simulink model "B4_quadcopter_model_discrete"  (R2021b)
settings: Solver=VariableStepAuto  StartTime=0.0  StopTime=10  FixedStep=0.002  RelTol=1e-3
values from neighbouring files (symbols this model uses):
  coef_sim_1 = tf_des_d.Denominator{1}(2)    [A11_setup_script_pprz.m]    (also in A1_setup_script.m; A6_slow_actuator.m)
  coef_sim_2 = tf_des_d.Numerator{1}(2)    [A11_setup_script_pprz.m]    (also in A1_setup_script.m; A6_slow_actuator.m)
  doublet_mag = - 0.15    (= -0.15)    [A11_setup_script_pprz.m]    (also in A1_setup_script.m)
  doublet_time = 6    [A11_setup_script_pprz.m]    (also in A1_setup_script.m)
  f_8 = 1    [A11_setup_script_pprz.m]    (also in A1_setup_script.m)
  FILT_CUTOFF = 2*pi*5    (= 31.4159265359)    [A11_setup_script_pprz.m]    (also in A1_setup_script.m)
  FILTER = 1    [A11_setup_script_pprz.m]    (also in A1_setup_script.m)
  G1 = inv(I)*G1_r    [A10_simple_plant.m]    (also in A11_setup_script_pprz.m = G1/scale; A1_setup_script.m = [G1;G1_T])
  G1_simple = inv(I)*G1_r_simple    [A1_setup_script.m]
  G2 = G2/scale    [A11_setup_script_pprz.m]    (also in A1_setup_script.m = (1/sampling_time)*inv(I)*(G2_r))
  h_plate = 0.3    [A11_setup_script_pprz.m]    (also in A1_setup_script.m = 0.16)
  I = eye(3,3)    [A10_simple_plant.m]    (also in A11_setup_script_pprz.m; A1_setup_script.m; A2_B_matrix_generation_symbolic.m = [Ixx 0 0; A3_B_matrix_generation_symbolic_cascaded.m = [Ixx 0 0)
  Iyy = 0.0008    [A11_setup_script_pprz.m]    (also in A1_setup_script.m = 0.0015)
  Izz = 0.000498    [A11_setup_script_pprz.m]    (also in A1_setup_script.m = 0.00015)
  K = 7    [A11_setup_script_pprz.m]    (also in A1_setup_script.m = 10)
  K_act = 50    [A10_simple_plant.m]    (also in A11_setup_script_pprz.m = 20; A1_setup_script.m = 20)
  K_act_outer = diag([K K K_act])    [A1_setup_script.m]
  K_d = 15    [A11_setup_script_pprz.m]    (also in A1_setup_script.m = 25)
  K_dd = K_act    (= 20)    [A11_setup_script_pprz.m]    (also in A1_setup_script.m)
  K_dyn = K    (= 10)    [A1_setup_script.m]
  K_ec = 50    [A11_setup_script_pprz.m]    (also in A1_setup_script.m = 251)
  K_ec_d = 13    [A11_setup_script_pprz.m]    (also in A1_setup_script.m = 25)
  K_ec_d_u = 1.5    [A11_setup_script_pprz.m]    (also in A1_setup_script.m = 5)
  K_ec_d_v = 1.5    [A11_setup_script_pprz.m]    (also in A1_setup_script.m = 5)
  K_ec_d_w = 1.5    [A11_setup_script_pprz.m]    (also in A1_setup_script.m = 5)
  K_ec_dd = 9    [A11_setup_script_pprz.m]    (also in A1_setup_script.m = 45)
  K_ec_i = 0    [A11_setup_script_pprz.m]    (also in A1_setup_script.m = 380)
  K_ec_u = 1.5    [A11_setup_script_pprz.m]    (also in A1_setup_script.m = 5)
  K_ec_v = 1.5    [A11_setup_script_pprz.m]    (also in A1_setup_script.m = 5)
  K_ec_w = 1.5    [A11_setup_script_pprz.m]    (also in A1_setup_script.m = 5)
  K_t = 0.0005    [A10_simple_plant.m]    (also in A11_setup_script_pprz.m = 6.557e-08; A1_setup_script.m = 6.557e-08)
  K_u = 1.0    (= 1)    [A11_setup_script_pprz.m]    (also in A1_setup_script.m = 1.5)
  K_u_d = 2.5    [A11_setup_script_pprz.m]    (also in A1_setup_script.m = 7)
  K_u_dd = K    (= 10)    [A1_setup_script.m]
  K_v = 1.0    (= 1)    [A11_setup_script_pprz.m]    (also in A1_setup_script.m = 1.5)
  K_v_d = 2.5    [A11_setup_script_pprz.m]    (also in A1_setup_script.m = 7)
  K_v_dd = K    (= 10)    [A1_setup_script.m]
  K_w = 1.0    (= 1)    [A11_setup_script_pprz.m]    (also in A1_setup_script.m = 4.5)
  K_w_d = 2.5    [A11_setup_script_pprz.m]    (also in A1_setup_script.m = 7)
  K_w_dd = K    (= 10)    [A1_setup_script.m]
  l_plate = 0.1    [A11_setup_script_pprz.m]    (also in A1_setup_script.m = 0.11)
  m = 0.4    [A10_simple_plant.m]    (also in A11_setup_script_pprz.m; A1_setup_script.m)
  NOISE = 0    [A11_setup_script_pprz.m]    (also in A1_setup_script.m)
  NOISE_ACC = 0.00005    (= 5e-05)    [A11_setup_script_pprz.m]    (also in A1_setup_script.m)
  NOISE_GYRO = 0.00005    (= 5e-05)    [A11_setup_script_pprz.m]    (also in A1_setup_script.m)
  NOISE_RPM = 200    [A11_setup_script_pprz.m]    (also in A1_setup_script.m)
  omega_act = 50    [A6_slow_actuator.m]
  omega_des = 20.00    (= 20)    [A11_setup_script_pprz.m]    (also in A1_setup_script.m; A6_slow_actuator.m = 49)
  sampling_time = 1/frequency    (= 0.002)    [A11_setup_script_pprz.m]    (also in A12_sim_multi_run.m; A1_setup_script.m; A6_slow_actuator.m)
  scale_8 = 1.6    [A11_setup_script_pprz.m]    (also in A1_setup_script.m)
  start_8 = 2    [A11_setup_script_pprz.m]    (also in A1_setup_script.m)
  start_time = 2    [A11_setup_script_pprz.m]    (also in A1_setup_script.m = 1)
  t_8 = 10    [A11_setup_script_pprz.m]    (also in A1_setup_script.m)
  w_plate = 0.3    [A11_setup_script_pprz.m]    (also in A1_setup_script.m = 0.36)
undefined symbols (not defined in the file or in its folder): DiscIntNeverNeededParam, K_ec_d_p, K_ec_d_q, K_ec_d_r, K_ec_dd_p, K_ec_dd_q, K_ec_dd_r, K_ec_i_u, K_ec_i_v, K_ec_i_w, K_ec_p, K_ec_q, K_ec_r, K_p, K_p_d, K_p_dd, K_q, K_q_d, K_q_dd, K_r, K_r_d, K_r_dd
libraries: simulink x44, cstblocks x37, dspinverses x26, dspmathops x9, dspstat3 x9, aerolibutil x9, sharedutil x3, aerolibanim x1
(part 1 of 13)
settings Model: Creator=pcampolucci  LastModifiedBy=pcampolucci

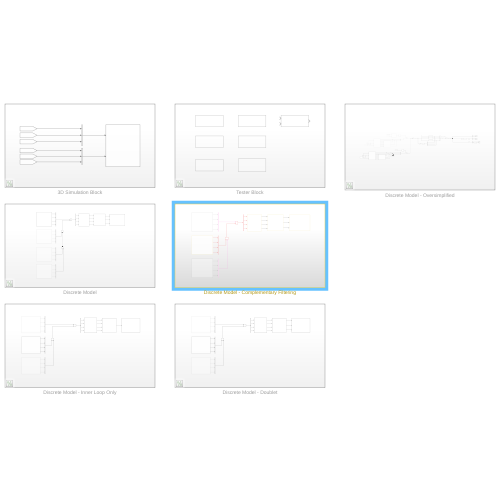
[thumbnail: Simulink's stored preview of the top-level diagram]
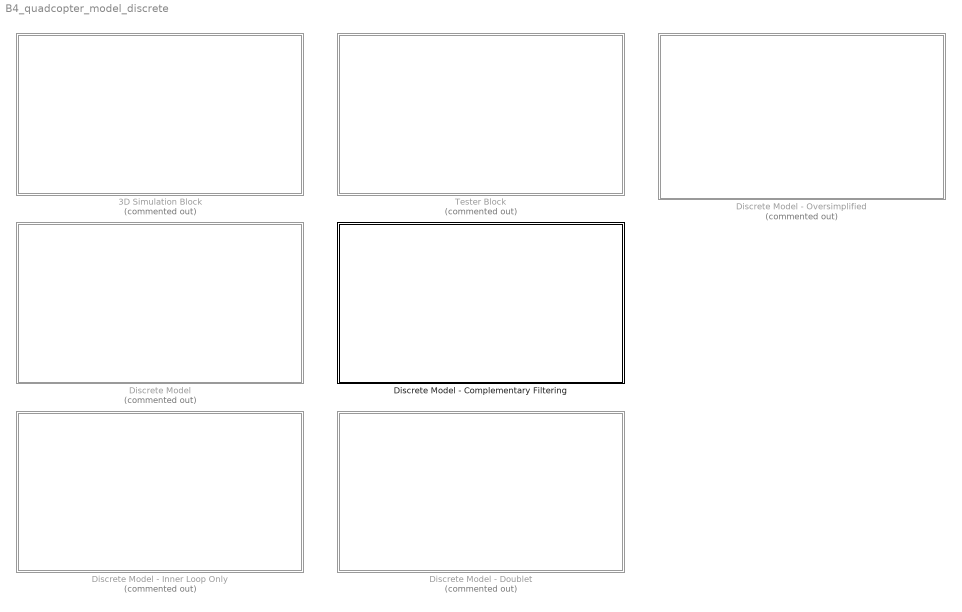
== system B4_quadcopter_model_discrete ==
  3D Simulation Block : Subsystem  Commented=on
  Discrete Model : Subsystem  Commented=on
  Discrete Model - Complementary Filtering : Subsystem
  Discrete Model - Doublet : Subsystem  Commented=on
  Discrete Model - Inner Loop Only : Subsystem  Commented=on
  Discrete Model - Oversimplified : Subsystem  Commented=on
  Tester Block : Subsystem  Commented=on

== system B4_quadcopter_model_discrete/3D Simulation Block ==
  6DoF Animation : aerolibanim/6DoF Animation  u1=[-4 4 -4 4 -1 1]  u2=0.02  u3=0.3  u4=[0 0 0]  u5=Fly alongside  u6=[5 5 -4]  u7=10  u8=on
  Vector Concatenate : Concatenate  NumInputs=3
  Vector Concatenate1 : Concatenate  NumInputs=3
  wires:
  [psi] -> Vector Concatenate/3
  Vector Concatenate1/1 -> 6DoF Animation/1
  Vector Concatenate/1 -> 6DoF Animation/2
  [X_cont] -> Vector Concatenate1/1
  [Y_cont] -> Vector Concatenate1/2
  [theta] -> Vector Concatenate/2
  [phi] -> Vector Concatenate/1
  [Z_cont] -> Vector Concatenate1/3

== system B4_quadcopter_model_discrete/Discrete Model ==
  Continuous Actuator Dynamics : Subsystem
  Demux : Demux
  Discrete INDI Controller Cascaded : Subsystem
  Discrete INDI Controller Cascaded w/ Actuator Compensation : Subsystem  Commented=on
  Discrete INDI Controller Cascaded w/ Actuator Compensation Double : Subsystem  Commented=on
  Discrete INDI Controller Cascaded w/ Actuator Compensation1 : Subsystem  Commented=on
  Force and Moment Calculation : Subsystem
      mask Display: image('C:\Users\pieca\Desktop\asc-indi-simulator\media\bebop.jpg'); % Use "Edit Image" on toolstrip to change.
  Manual Switch1 : ManualSwitch
  Manual Switch2 : ManualSwitch
  Manual Switch3 : ManualSwitch
  Mux{1,3..5} (4 alike) : Mux
  Plant and State Estimation : Subsystem
  wires:
  Demux/2 -> Continuous Actuator Dynamics/2(Motor_2_omega_input)
  Demux/4 -> Continuous Actuator Dynamics/4(Motor_4_omega_input)
  Continuous Actuator Dynamics/1(omega_1) -> Force and Moment Calculation/1(omega_1)
  Continuous Actuator Dynamics/4(omega_4) -> Force and Moment Calculation/4(omega_4)
  Demux/1 -> Continuous Actuator Dynamics/1(Motor_1_omega_input)
  Force and Moment Calculation/1(Moments in body frame) -> Plant and State Estimation/1(Moments in body frame)
  Continuous Actuator Dynamics/3(omega_3) -> Force and Moment Calculation/3(omega_3)
  Continuous Actuator Dynamics/2(omega_2) -> Force and Moment Calculation/2(omega_2)
  Manual Switch2/1 -> Demux/1
  Demux/3 -> Continuous Actuator Dynamics/3(Motor_3_omega_input)
  Discrete INDI Controller Cascaded/2(Motor_2_omega_input) -> Mux3/2
  Discrete INDI Controller Cascaded/3(Motor_3_omega_input) -> Mux3/3
  Discrete INDI Controller Cascaded/4(Motor_4_omega_input) -> Mux3/4
  Discrete INDI Controller Cascaded/1(Motor_1_omega_input) -> Mux3/1
  Force and Moment Calculation/2(Forces in earth frame) -> Plant and State Estimation/2(Forces in earth frame)
  Discrete INDI Controller Cascaded w/ Actuator Compensation/2(Motor_2_omega_input) -> Mux4/2
  Discrete INDI Controller Cascaded w/ Actuator Compensation/1(Motor_1_omega_input) -> Mux4/1
  Discrete INDI Controller Cascaded w/ Actuator Compensation/3(Motor_3_omega_input) -> Mux4/3
  Discrete INDI Controller Cascaded w/ Actuator Compensation/4(Motor_4_omega_input) -> Mux4/4
  Mux3/1 -> Manual Switch2/1
  Force and Moment Calculation/3(Collective Thrust) -> Plant and State Estimation/3(Collective Thrust)
  Mux4/1 -> Manual Switch3/1
  Manual Switch3/1 -> Manual Switch2/2
  Discrete INDI Controller Cascaded w/ Actuator Compensation Double/4(Motor_4_omega_input) -> Mux5/4
  Discrete INDI Controller Cascaded w/ Actuator Compensation Double/3(Motor_3_omega_input) -> Mux5/3
  Discrete INDI Controller Cascaded w/ Actuator Compensation Double/1(Motor_1_omega_input) -> Mux5/1
  Discrete INDI Controller Cascaded w/ Actuator Compensation Double/2(Motor_2_omega_input) -> Mux5/2
  Discrete INDI Controller Cascaded w/ Actuator Compensation1/1(Motor_1_omega_input) -> Mux1/1
  Discrete INDI Controller Cascaded w/ Actuator Compensation1/4(Motor_4_omega_input) -> Mux1/4
  Discrete INDI Controller Cascaded w/ Actuator Compensation1/2(Motor_2_omega_input) -> Mux1/2
  Discrete INDI Controller Cascaded w/ Actuator Compensation1/3(Motor_3_omega_input) -> Mux1/3
  Mux1/1 -> Manual Switch1/1
  Manual Switch1/1 -> Manual Switch3/2
  Mux5/1 -> Manual Switch1/2

== system B4_quadcopter_model_discrete/Discrete Model - Complementary Filtering ==
  Continuous Actuator Dynamics : Subsystem
  Demux : Demux
  Discrete INDI Controller Cascaded : Subsystem  Commented=on
  Discrete INDI Controller Cascaded w/ Actuator Compensation : Subsystem
  Discrete INDI Controller Cascaded w/ Actuator Compensation Double : Subsystem  Commented=on
  Force and Moment Calculation : Subsystem
      mask Display: image('/home/pcampolucci/asc-indi-simulator/media/bebop.jpg'); % Use "Edit Image" on toolstrip to change.
  Manual Switch2 : ManualSwitch  CurrentSetting=0
  Manual Switch3 : ManualSwitch
  Mux3 : Mux
  Mux4 : Mux
  Mux5 : Mux
  Plant and State Estimation : Subsystem
  wires:
  Demux/2 -> Continuous Actuator Dynamics/2(Motor_2_omega_input)
  Demux/4 -> Continuous Actuator Dynamics/4(Motor_4_omega_input)
  Continuous Actuator Dynamics/1(omega_1) -> Force and Moment Calculation/1(omega_1)
  Continuous Actuator Dynamics/4(omega_4) -> Force and Moment Calculation/4(omega_4)
  Demux/1 -> Continuous Actuator Dynamics/1(Motor_1_omega_input)
  Force and Moment Calculation/1(Moments in body frame) -> Plant and State Estimation/1(Moments in body frame)
  Continuous Actuator Dynamics/3(omega_3) -> Force and Moment Calculation/3(omega_3)
  Continuous Actuator Dynamics/2(omega_2) -> Force and Moment Calculation/2(omega_2)
  Manual Switch2/1 -> Demux/1
  Demux/3 -> Continuous Actuator Dynamics/3(Motor_3_omega_input)
  Discrete INDI Controller Cascaded/2(Motor_2_omega_input) -> Mux3/2
  Discrete INDI Controller Cascaded/3(Motor_3_omega_input) -> Mux3/3
  Discrete INDI Controller Cascaded/4(Motor_4_omega_input) -> Mux3/4
  Discrete INDI Controller Cascaded/1(Motor_1_omega_input) -> Mux3/1
  Force and Moment Calculation/2(Forces in earth frame) -> Plant and State Estimation/2(Forces in earth frame)
  Discrete INDI Controller Cascaded w/ Actuator Compensation/2(Motor_2_omega_input) -> Mux4/2
  Discrete INDI Controller Cascaded w/ Actuator Compensation/1(Motor_1_omega_input) -> Mux4/1
  Discrete INDI Controller Cascaded w/ Actuator Compensation/3(Motor_3_omega_input) -> Mux4/3
  Discrete INDI Controller Cascaded w/ Actuator Compensation/4(Motor_4_omega_input) -> Mux4/4
  Mux3/1 -> Manual Switch2/1
  Force and Moment Calculation/3(Collective Thrust) -> Plant and State Estimation/3(Collective Thrust)
  Mux4/1 -> Manual Switch3/1
  Manual Switch3/1 -> Manual Switch2/2
  Discrete INDI Controller Cascaded w/ Actuator Compensation Double/4(Motor_4_omega_input) -> Mux5/4
  Discrete INDI Controller Cascaded w/ Actuator Compensation Double/3(Motor_3_omega_input) -> Mux5/3
  Discrete INDI Controller Cascaded w/ Actuator Compensation Double/1(Motor_1_omega_input) -> Mux5/1
  Discrete INDI Controller Cascaded w/ Actuator Compensation Double/2(Motor_2_omega_input) -> Mux5/2
  Mux5/1 -> Manual Switch3/2

== system B4_quadcopter_model_discrete/Discrete Model - Doublet ==
  Continuous Actuator Dynamics : Subsystem
  Demux : Demux
  Discrete INDI Controller Cascaded : Subsystem  Commented=on
  Discrete INDI Controller Cascaded w/ Actuator Compensation : Subsystem
  Discrete INDI Controller Cascaded w/ Actuator Compensation Double : Subsystem  Commented=on
  Force and Moment Calculation : Subsystem
      mask Display: image('C:\Users\pieca\Desktop\asc-indi-simulator\media\bebop.jpg'); % Use "Edit Image" on toolstrip to change.
  Manual Switch2 : ManualSwitch  CurrentSetting=0
  Manual Switch3 : ManualSwitch
  Mux3 : Mux
  Mux4 : Mux
  Mux5 : Mux
  Plant and State Estimation : Subsystem
  wires:
  Demux/2 -> Continuous Actuator Dynamics/2(Motor_2_omega_input)
  Demux/4 -> Continuous Actuator Dynamics/4(Motor_4_omega_input)
  Continuous Actuator Dynamics/1(omega_1) -> Force and Moment Calculation/1(omega_1)
  Continuous Actuator Dynamics/4(omega_4) -> Force and Moment Calculation/4(omega_4)
  Demux/1 -> Continuous Actuator Dynamics/1(Motor_1_omega_input)
  Force and Moment Calculation/1(Moments in body frame) -> Plant and State Estimation/1(Moments in body frame)
  Continuous Actuator Dynamics/3(omega_3) -> Force and Moment Calculation/3(omega_3)
  Continuous Actuator Dynamics/2(omega_2) -> Force and Moment Calculation/2(omega_2)
  Manual Switch2/1 -> Demux/1
  Demux/3 -> Continuous Actuator Dynamics/3(Motor_3_omega_input)
  Discrete INDI Controller Cascaded/2(Motor_2_omega_input) -> Mux3/2
  Discrete INDI Controller Cascaded/3(Motor_3_omega_input) -> Mux3/3
  Discrete INDI Controller Cascaded/4(Motor_4_omega_input) -> Mux3/4
  Discrete INDI Controller Cascaded/1(Motor_1_omega_input) -> Mux3/1
  Force and Moment Calculation/2(Forces in earth frame) -> Plant and State Estimation/2(Forces in earth frame)
  Discrete INDI Controller Cascaded w/ Actuator Compensation/2(Motor_2_omega_input) -> Mux4/2
  Discrete INDI Controller Cascaded w/ Actuator Compensation/1(Motor_1_omega_input) -> Mux4/1
  Discrete INDI Controller Cascaded w/ Actuator Compensation/3(Motor_3_omega_input) -> Mux4/3
  Discrete INDI Controller Cascaded w/ Actuator Compensation/4(Motor_4_omega_input) -> Mux4/4
  Mux3/1 -> Manual Switch2/1
  Force and Moment Calculation/3(Collective Thrust) -> Plant and State Estimation/3(Collective Thrust)
  Mux4/1 -> Manual Switch3/1
  Manual Switch3/1 -> Manual Switch2/2
  Discrete INDI Controller Cascaded w/ Actuator Compensation Double/4(Motor_4_omega_input) -> Mux5/4
  Discrete INDI Controller Cascaded w/ Actuator Compensation Double/3(Motor_3_omega_input) -> Mux5/3
  Discrete INDI Controller Cascaded w/ Actuator Compensation Double/1(Motor_1_omega_input) -> Mux5/1
  Discrete INDI Controller Cascaded w/ Actuator Compensation Double/2(Motor_2_omega_input) -> Mux5/2
  Mux5/1 -> Manual Switch3/2

== system B4_quadcopter_model_discrete/Discrete Model - Inner Loop Only ==
  Continuous Actuator Dynamics : Subsystem
  Demux : Demux
  Discrete INDI Controller Cascaded : Subsystem  Commented=on
  Discrete INDI Controller Cascaded w/ Actuator Compensation : Subsystem
  Discrete INDI Controller Cascaded w/ Actuator Compensation Double : Subsystem  Commented=on
  Force and Moment Calculation : Subsystem
      mask Display: image('C:\Users\pieca\Desktop\asc-indi-simulator\media\bebop.jpg'); % Use "Edit Image" on toolstrip to change.
  Manual Switch2 : ManualSwitch  CurrentSetting=0
  Manual Switch3 : ManualSwitch
  Mux3 : Mux
  Mux4 : Mux
  Mux5 : Mux
  Plant and State Estimation : Subsystem
  wires:
  Demux/2 -> Continuous Actuator Dynamics/2(Motor_2_omega_input)
  Demux/4 -> Continuous Actuator Dynamics/4(Motor_4_omega_input)
  Continuous Actuator Dynamics/1(omega_1) -> Force and Moment Calculation/1(omega_1)
  Continuous Actuator Dynamics/4(omega_4) -> Force and Moment Calculation/4(omega_4)
  Demux/1 -> Continuous Actuator Dynamics/1(Motor_1_omega_input)
  Force and Moment Calculation/1(Moments in body frame) -> Plant and State Estimation/1(Moments in body frame)
  Continuous Actuator Dynamics/3(omega_3) -> Force and Moment Calculation/3(omega_3)
  Continuous Actuator Dynamics/2(omega_2) -> Force and Moment Calculation/2(omega_2)
  Manual Switch2/1 -> Demux/1
  Demux/3 -> Continuous Actuator Dynamics/3(Motor_3_omega_input)
  Discrete INDI Controller Cascaded/2(Motor_2_omega_input) -> Mux3/2
  Discrete INDI Controller Cascaded/3(Motor_3_omega_input) -> Mux3/3
  Discrete INDI Controller Cascaded/4(Motor_4_omega_input) -> Mux3/4
  Discrete INDI Controller Cascaded/1(Motor_1_omega_input) -> Mux3/1
  Discrete INDI Controller Cascaded w/ Actuator Compensation/2(Motor_2_omega_input) -> Mux4/2
  Discrete INDI Controller Cascaded w/ Actuator Compensation/1(Motor_1_omega_input) -> Mux4/1
  Discrete INDI Controller Cascaded w/ Actuator Compensation/3(Motor_3_omega_input) -> Mux4/3
  Discrete INDI Controller Cascaded w/ Actuator Compensation/4(Motor_4_omega_input) -> Mux4/4
  Mux3/1 -> Manual Switch2/1
  Mux4/1 -> Manual Switch3/1
  Manual Switch3/1 -> Manual Switch2/2
  Discrete INDI Controller Cascaded w/ Actuator Compensation Double/4(Motor_4_omega_input) -> Mux5/4
  Discrete INDI Controller Cascaded w/ Actuator Compensation Double/3(Motor_3_omega_input) -> Mux5/3
  Discrete INDI Controller Cascaded w/ Actuator Compensation Double/1(Motor_1_omega_input) -> Mux5/1
  Discrete INDI Controller Cascaded w/ Actuator Compensation Double/2(Motor_2_omega_input) -> Mux5/2
  Mux5/1 -> Manual Switch3/2

== system B4_quadcopter_model_discrete/Discrete Model - Oversimplified ==
  Butterworth Lowpass 2nd Order1 : Subsystem
  Butterworth Lowpass 2nd Order4 : Subsystem
  Constant : Constant  Commented=on  Value=0
  Constant1 : Constant  Value=G1_simple  SampleTime=sampling_time
  Constant2 : Constant  Commented=on  Value=G1_simple  SampleTime=sampling_time
  Constant3 : Constant  Value=0
  Constant4 : Constant  Value=G1_simple  SampleTime=sampling_time
  Constant6 : Constant  Commented=on  Value=K_act  SampleTime=sampling_time
  Delay : Delay  DelayLength=1  SampleTime=sampling_time
  Delay1 : Delay  DelayLength=1  SampleTime=sampling_time
  Demux : Demux
  Demux3 : Demux  Outputs=3
  Demux4 : Demux  Outputs=3
  Demux5 : Demux  Outputs=3
  Discrete Derivative : simulink/Discrete/Discrete Derivative  gainval=1.0  ICPrevScaledInput=0.0  OutMin=[]  OutMax=[]  OutDataType=fixdt(1, 16)  OutScaling=2^-10  DoSatur=off
  Discrete-Time Integrator : DiscreteIntegrator  SampleTime=sampling_time  ICPrevOutput=DiscIntNeverNeededParam  ICPrevScaledInput=DiscIntNeverNeededParam
  Doublet Block : Subsystem  Commented=on
  Doublet Block1 : Subsystem
  ERROR CONTROLLER ATTITUDE : Subsystem  Commented=on
  ERROR CONTROLLER ATTITUDE1 : Subsystem
  G1+G2 : MATLAB Function  Commented=on  TreatAsAtomicUnit=on
  Gyro : ZeroOrderHold  SampleTime=sampling_time
  INTERNAL REFERENCE MODEL ATTITUDE : Subsystem  Commented=on
  INTERNAL REFERENCE MODEL ATTITUDE1 : Subsystem
  Integrator : Integrator
  Manual Switch : ManualSwitch  CurrentSetting=0
  Matrix Multiply : Product  Commented=on  Multiplication=Matrix(*)
  Matrix Multiply1 : Product  Multiplication=Matrix(*)
  Matrix Multiply2 : Product  Multiplication=Matrix(*)
  Mux : Mux
  Pseudoinverse1 : dspinverses/Pseudoinverse  wanterr=off  SimulateUsing=Interpreted execution
      settings: SourceProductBaseCode=DS
  Pseudoinverse2 : dspinverses/Pseudoinverse  Commented=on  wanterr=off  SimulateUsing=Interpreted execution
      settings: SourceProductBaseCode=DS
  Sum{1,4,11,13} (4 alike) : Sum  Commented=on  Inputs=|++
  Sum{2,5..6,8,10} (5 alike) : Sum  Inputs=|++
  Sum3 : Sum  Inputs=|+-
  Sum7 : Sum  Inputs=|+-
  Sum9 : Sum  Inputs=|+-
  Transfer Fcn{,1..3} (4 alike) : TransferFcn  Numerator=[omega_des]  Denominator=[1 omega_des]
  Vector Concatenate : Concatenate  Commented=on  NumInputs=3
  Vector Concatenate1 : Concatenate  NumInputs=4
  Vector Concatenate2 : Concatenate  NumInputs=3
  wrapper : MATLAB Function  TreatAsAtomicUnit=on
  tag scope: p=global, pd_f=global, phi=global, psi=global, q=global, qd_f=global, r=global, rd_f=global, theta=global
  wires:
  INTERNAL REFERENCE MODEL ATTITUDE/12(psi_ref) -> ERROR CONTROLLER ATTITUDE/9(psi_ref)
  Sum11/1 -> Vector Concatenate/2  "qdd_des"
  Constant/1 -> INTERNAL REFERENCE MODEL ATTITUDE/3(psi_cmd), INTERNAL REFERENCE MODEL ATTITUDE/1(phi_cmd), Sum1/1  "phi_cmd"
  Pseudoinverse2/1 -> Matrix Multiply/1
  INTERNAL REFERENCE MODEL ATTITUDE/8(q_ref) -> ERROR CONTROLLER ATTITUDE/5(q_ref)
  INTERNAL REFERENCE MODEL ATTITUDE/7(p_ref) -> ERROR CONTROLLER ATTITUDE/4(p_ref)
  INTERNAL REFERENCE MODEL ATTITUDE/11(theta_ref) -> ERROR CONTROLLER ATTITUDE/8(theta_ref)
  Matrix Multiply/1 -> Manual Switch/1  "du"
  Doublet Block/1(Out1) -> Sum1/2
  Sum4/1 -> Vector Concatenate/1  "pdd_des"
  G1+G2/1(B_inner) -> Pseudoinverse2/1  "B_inner"
  Vector Concatenate1/1 -> Butterworth Lowpass 2nd Order1/1(In)  "u"
  ERROR CONTROLLER ATTITUDE/3(rdd_ec) -> Sum13/2  "rdd_ec"
  ERROR CONTROLLER ATTITUDE/1(pdd_ec) -> Sum4/2  "pdd_ec"
  INTERNAL REFERENCE MODEL ATTITUDE/5(qd_ref) -> ERROR CONTROLLER ATTITUDE/2(qd_ref)
  INTERNAL REFERENCE MODEL ATTITUDE/10(phi_ref) -> ERROR CONTROLLER ATTITUDE/7(phi_ref)
  INTERNAL REFERENCE MODEL ATTITUDE/3(rdd_ref) -> Sum13/1
  Constant6/1 -> G1+G2/2(K_act)
  INTERNAL REFERENCE MODEL ATTITUDE/6(rd_ref) -> ERROR CONTROLLER ATTITUDE/3(rd_ref)
  INTERNAL REFERENCE MODEL ATTITUDE/1(pdd_ref) -> Sum4/1
  ERROR CONTROLLER ATTITUDE/2(qdd_ec) -> Sum11/2  "qdd_ec"
  Sum1/1 -> INTERNAL REFERENCE MODEL ATTITUDE/2(theta_cmd)  "theta_cmd"
  Constant2/1 -> G1+G2/1(G1_simple)
  INTERNAL REFERENCE MODEL ATTITUDE/4(pd_ref) -> ERROR CONTROLLER ATTITUDE/1(pd_ref)
  INTERNAL REFERENCE MODEL ATTITUDE/9(r_ref) -> ERROR CONTROLLER ATTITUDE/6(r_ref)
  INTERNAL REFERENCE MODEL ATTITUDE/2(qdd_ref) -> Sum11/1
  Sum13/1 -> Vector Concatenate/3  "rdd_des"
  Sum8/1 -> Demux/1  "u_cmd"
  Vector Concatenate/1 -> Matrix Multiply/2
  Demux/4 -> Transfer Fcn3/1  "omega_4_in"
  Transfer Fcn/1 -> Mux/1, Vector Concatenate1/1  "omega_1"
  Transfer Fcn1/1 -> Mux/2, Vector Concatenate1/2  "omega_2"
  Demux/3 -> Transfer Fcn2/1  "omega_3_in"
  Transfer Fcn3/1 -> Mux/4, Vector Concatenate1/4  "omega_4"
  Transfer Fcn2/1 -> Mux/3, Vector Concatenate1/3  "omega_3"
  Demux/2 -> Transfer Fcn1/1  "omega_2_in"
  Demux/1 -> Transfer Fcn/1  "omega_1_in"
  Mux/1 -> Matrix Multiply1/2
  Constant1/1 -> Matrix Multiply1/1
  wrapper/1(psie_w) -> [psi]  "psi"
  Demux5/1 -> [p]  "p"
  Gyro/1 -> Delay1/1, Discrete-Time Integrator/1, Demux5/1  "pqr_measured"
  Demux3/2 -> [theta]  "theta"
  Demux4/2 -> [qd_f]  "qd_f"
  Demux4/3 -> [rd_f]  "rd_f"
  Discrete-Time Integrator/1 -> Demux3/1
  Demux4/1 -> [pd_f]  "pd_f"
  Demux5/3 -> [r]  "r"
  Delay1/1 -> Butterworth Lowpass 2nd Order4/1(In)
  Butterworth Lowpass 2nd Order4/1(Out) -> Discrete Derivative/1
  Demux3/3 -> wrapper/1(pis_e)
  Demux3/1 -> [phi]  "phi"
  Demux5/2 -> [q]  "q"
  Matrix Multiply1/1 -> Integrator/1
  Integrator/1 -> Gyro/1
  Delay/1 -> Sum8/2
  Constant3/1 -> INTERNAL REFERENCE MODEL ATTITUDE1/3(psi_cmd), INTERNAL REFERENCE MODEL ATTITUDE1/1(phi_cmd), Sum2/1  "phi_cmd"
  Constant4/1 -> Pseudoinverse1/1  "B_inner"
  Pseudoinverse1/1 -> Matrix Multiply2/1
  Vector Concatenate2/1 -> Matrix Multiply2/2
  Doublet Block1/1(Out1) -> Sum2/2
  Matrix Multiply2/1 -> Manual Switch/2  "du"
  Sum3/1 -> Vector Concatenate2/1
  ERROR CONTROLLER ATTITUDE1/1(pd_ec) -> Sum10/2  "pd_ec"
  INTERNAL REFERENCE MODEL ATTITUDE1/4(p_ref) -> ERROR CONTROLLER ATTITUDE1/1(p_ref)  "p_ref"
  INTERNAL REFERENCE MODEL ATTITUDE1/6(r_ref) -> ERROR CONTROLLER ATTITUDE1/3(r_ref)  "r_ref"
  [rd_f] -> Sum9/2
  INTERNAL REFERENCE MODEL ATTITUDE1/5(q_ref) -> ERROR CONTROLLER ATTITUDE1/2(q_ref)  "q_ref"
  Sum5/1 -> Sum7/1  "qd_des"
  INTERNAL REFERENCE MODEL ATTITUDE1/9(psi_ref) -> ERROR CONTROLLER ATTITUDE1/6(psi_ref)  "psi_ref"
  INTERNAL REFERENCE MODEL ATTITUDE1/2(qd_ref) -> Sum5/1  "qd_ref"
  [qd_f] -> Sum7/2
  INTERNAL REFERENCE MODEL ATTITUDE1/1(pd_ref) -> Sum10/1  "pd_ref"
  ERROR CONTROLLER ATTITUDE1/2(qd_ec) -> Sum5/2  "qd_ec"
  Sum7/1 -> Vector Concatenate2/2
  ERROR CONTROLLER ATTITUDE1/3(rd_ec) -> Sum6/2  "rd_ec"
  Sum9/1 -> Vector Concatenate2/3
  INTERNAL REFERENCE MODEL ATTITUDE1/8(theta_ref) -> ERROR CONTROLLER ATTITUDE1/5(theta_ref)  "theta_ref"
  [pd_f] -> Sum3/2
  INTERNAL REFERENCE MODEL ATTITUDE1/3(rd_ref) -> Sum6/1  "rd_ref"
  Sum10/1 -> Sum3/1  "pd_des"
  INTERNAL REFERENCE MODEL ATTITUDE1/7(phi_ref) -> ERROR CONTROLLER ATTITUDE1/4(phi_ref)  "phi_ref"
  Sum6/1 -> Sum9/1  "rd_des"
  Sum2/1 -> INTERNAL REFERENCE MODEL ATTITUDE1/2(theta_cmd)  "theta_cmd"
  Discrete Derivative/1 -> Demux4/1
  Manual Switch/1 -> Sum8/1
  Butterworth Lowpass 2nd Order1/1(Out) -> Delay/1

== system B4_quadcopter_model_discrete/Tester Block ==
  8-shaped trajectory : Subsystem  Commented=on
  Complementary Filter : Subsystem  Commented=on
  Slowdown Actuator : Subsystem  Commented=on
  Tester Actuator State Estimator : Subsystem  Commented=on
  Tester RM and EC : Subsystem  Commented=on
  Tester State Estimator : Subsystem  Commented=on
  Wrapping Test : Subsystem  Commented=on

== system B4_quadcopter_model_discrete/Discrete Model/Continuous Actuator Dynamics ==
  Motor_1_omega_input : Inport
  Motor_2_omega_input : Inport  Port=2
  Motor_3_omega_input : Inport  Port=3
  Motor_4_omega_input : Inport  Port=4
  Butterworth Lowpass 2nd Order1 : Subsystem
  Demux : Demux
  Discrete Transfer Fcn{1..4} (4 alike) : DiscreteTransferFcn  Numerator=[coef_sim_2]  Denominator=[1 coef_sim_1]  SampleTime=sampling_time
  Mux : Mux
  RPM Noise : simulink/Sources/Band-Limited White Noise  Cov=[NOISE_RPM]  Ts=sampling_time  seed=[23341]
  Saturation{,1..3} (4 alike) : Saturate  UpperLimit=12000  LowerLimit=10
  Sum : Sum  Inputs=|++
  Transfer Fcn{,1..3} (4 alike) : TransferFcn  Numerator=[omega_des]  Denominator=[1 omega_des]
  omega_1 : Outport
  omega_2 : Outport  Port=2
  omega_3 : Outport  Port=3
  omega_4 : Outport  Port=4
  tag scope: omega_1_f=global, omega_2_f=global, omega_3_f=global, omega_4_f=global
  wires:
  Transfer Fcn3/1 -> omega_4/1  "omega_4"
  Motor_4_omega_input/1 -> Saturation3/1  "omega_4_in"
  Saturation/1 -> Discrete Transfer Fcn2/1, Transfer Fcn/1
  Motor_3_omega_input/1 -> Saturation2/1  "omega_3_in"
  Transfer Fcn1/1 -> omega_2/1  "omega_2"
  Saturation1/1 -> Transfer Fcn1/1, Discrete Transfer Fcn1/1
  Saturation3/1 -> Transfer Fcn3/1, Discrete Transfer Fcn4/1
  Discrete Transfer Fcn2/1 -> Mux/1
  Saturation2/1 -> Transfer Fcn2/1, Discrete Transfer Fcn3/1
  Motor_2_omega_input/1 -> Saturation1/1  "omega_2_in"
  Demux/2 -> [omega_2_f]  "omega_2_est"
  Motor_1_omega_input/1 -> Saturation/1  "omega_1_in"
  Transfer Fcn/1 -> omega_1/1  "omega_1"
  Demux/4 -> [omega_4_f]  "omega_4_est"
  Discrete Transfer Fcn4/1 -> Mux/4
  Discrete Transfer Fcn1/1 -> Mux/2
  Discrete Transfer Fcn3/1 -> Mux/3
  Transfer Fcn2/1 -> omega_3/1  "omega_3"
  Demux/1 -> [omega_1_f]  "omega_1_est"
  Demux/3 -> [omega_3_f]  "omega_3_est"
  Mux/1 -> Sum/1
  Butterworth Lowpass 2nd Order1/1(Out) -> Demux/1
  RPM Noise/1 -> ?
  Sum/1 -> Butterworth Lowpass 2nd Order1/1(In)

== system B4_quadcopter_model_discrete/Discrete Model/Discrete INDI Controller Cascaded ==
  note: Inner Loop
  note: Outer Loop
  8-shape trajectory : Subsystem
  Constant1 : Constant  Value=m  SampleTime=sampling_time
  Constant2 : Constant  Value=G1  SampleTime=sampling_time
  Constant3 : Constant  Value=G2  SampleTime=sampling_time
  Constant4 : Constant  Value=0
  Constant5 : Constant  Value=0
  Constant8 : Constant  Value=0  SampleTime=sampling_time
  Constant9 : Constant  Value=G2  SampleTime=sampling_time
  Demux : Demux
  Demux1 : Demux
  Demux5 : Demux  Outputs=3
  Discrete Transfer Fcn : DiscreteTransferFcn  Denominator=[1 0]
  Display : Display
  Display1 : Display
  ERROR CONTROLLER ATTITUDE : Subsystem
  ERROR CONTROLLER VELOCITY : Subsystem
  G1+G2 : MATLAB Function  TreatAsAtomicUnit=on
  G2_comp : MATLAB Function  TreatAsAtomicUnit=on
  INTERNAL REFERENCE MODEL ATTITUDE : Subsystem
  INTERNAL REFERENCE MODEL VELOCITY : Subsystem
  MATLAB Function1 : MATLAB Function  TreatAsAtomicUnit=on
  Matrix Multiply : Product  Multiplication=Matrix(*)
  MatrixMultiply1 : Product  Multiplication=Matrix(*)
  Pseudoinverse1 : dspinverses/Pseudoinverse  wanterr=off  SimulateUsing=Interpreted execution
      settings: SourceProductBaseCode=DS
  Pseudoinverse2 : dspinverses/Pseudoinverse  wanterr=off  SimulateUsing=Interpreted execution
      settings: SourceProductBaseCode=DS
  Saturation : Saturate
  Saturation1 : Saturate
  Saturation4 : Saturate  UpperLimit=12000  LowerLimit=10
  Scope{1,7,9,11} (4 alike) : Scope
  Sum{,4,6..8,11..13,16,20} (10 alike) : Sum  Inputs=|++
  Sum{1..3,17..19} (6 alike) : Sum  Inputs=|+-
  Sum15 : Sum  Inputs=|-+
  Sum21 : Sum  Inputs=|-+
  Vector Concatenate : Concatenate  NumInputs=4
  Vector Concatenate1 : Concatenate  NumInputs=4
  Vector Concatenate2 : Concatenate  NumInputs=4
  Vector Concatenate3 : Concatenate  NumInputs=3
  Motor_1_omega_input : Outport
  Motor_2_omega_input : Outport  Port=2
  Motor_3_omega_input : Outport  Port=3
  Motor_4_omega_input : Outport  Port=4
  tag scope: psi_traj=global
  wires:
  Sum13/1 -> Sum3/1  "rd_des"
  Sum4/1 -> Sum1/1  "pd_des"
  Sum2/1 -> Vector Concatenate/2
  ERROR CONTROLLER ATTITUDE/1(pd_ec) -> Sum4/2  "pd_ec"
  Sum3/1 -> Vector Concatenate/3
  ERROR CONTROLLER ATTITUDE/3(rd_ec) -> Sum13/2  "rd_ec"
  INTERNAL REFERENCE MODEL ATTITUDE/5(q_ref) -> ERROR CONTROLLER ATTITUDE/2(q_ref)  "q_ref"
  Vector Concatenate/1 -> [dv_inner], Scope1/1
  [pd_f] -> Sum1/2
  INTERNAL REFERENCE MODEL ATTITUDE/3(rd_ref) -> Sum13/1  "rd_ref"
  INTERNAL REFERENCE MODEL ATTITUDE/9(psi_ref) -> ERROR CONTROLLER ATTITUDE/6(psi_ref)  "psi_ref"
  INTERNAL REFERENCE MODEL ATTITUDE/4(p_ref) -> ERROR CONTROLLER ATTITUDE/1(p_ref)  "p_ref"
  INTERNAL REFERENCE MODEL ATTITUDE/6(r_ref) -> ERROR CONTROLLER ATTITUDE/3(r_ref)  "r_ref"
  INTERNAL REFERENCE MODEL ATTITUDE/8(theta_ref) -> ERROR CONTROLLER ATTITUDE/5(theta_ref)  "theta_ref"
  INTERNAL REFERENCE MODEL ATTITUDE/7(phi_ref) -> ERROR CONTROLLER ATTITUDE/4(phi_ref)  "phi_ref"
  ERROR CONTROLLER ATTITUDE/2(qd_ec) -> Sum11/2  "qd_ec"
  INTERNAL REFERENCE MODEL ATTITUDE/1(pd_ref) -> Sum4/1  "pd_ref"
  Sum1/1 -> Vector Concatenate/1
  Sum11/1 -> Sum2/1  "qd_des"
  [qd_f] -> Sum2/2
  INTERNAL REFERENCE MODEL ATTITUDE/2(qd_ref) -> Sum11/1  "qd_ref"
  [rd_f] -> Sum3/2
  [T_increment] -> Vector Concatenate/4
  Vector Concatenate3/1 -> Scope7/1, [dv_outer]
  Sum20/1 -> [Phi_cmd]  "phi_cmd"
  INTERNAL REFERENCE MODEL VELOCITY/5(Vy_ref) -> ERROR CONTROLLER VELOCITY/2(Vy_ref)  "Vy_ref"
  [Ax_f] -> Sum17/2
  Demux5/2 -> Sum20/1
  Sum19/1 -> Vector Concatenate3/3  "dv_z"
  8-shape trajectory/1(xd_traj) -> INTERNAL REFERENCE MODEL VELOCITY/1(Vx_cmd)  "Vx_cmd"
  Pseudoinverse1/1 -> Scope11/1, MatrixMultiply1/1
  MatrixMultiply1/1 -> Demux5/1  "du"
  MATLAB Function1/1(B_outer) -> Scope9/1, Display1/1, Pseudoinverse1/1
  Sum21/1 -> Sum16/2  "u"
  8-shape trajectory/2(yd_traj) -> INTERNAL REFERENCE MODEL VELOCITY/2(Vy_cmd)  "Vy_cmd"
  INTERNAL REFERENCE MODEL VELOCITY/3(Az_ref) -> Sum12/1  "Az_ref"
  Sum18/1 -> Vector Concatenate3/2  "dv_y"
  Sum6/1 -> Sum17/1
  [psi_f] -> MATLAB Function1/4(Psi)
  Sum15/1 -> Sum20/2  "u"
  Constant5/1 -> Sum15/1
  INTERNAL REFERENCE MODEL VELOCITY/2(Ay_ref) -> Sum7/1  "Ay_ref"
  Sum7/1 -> Sum18/1
  Constant8/1 -> INTERNAL REFERENCE MODEL VELOCITY/3(Vz_cmd)  "Vz_cmd"
  8-shape trajectory/3(psi_traj) -> [psi_traj]
  Demux5/3 -> [T_increment]  "t_incr"
  INTERNAL REFERENCE MODEL VELOCITY/1(Ax_ref) -> Sum6/1  "Ax_ref"
  Constant1/1 -> MATLAB Function1/5(m)
  ERROR CONTROLLER VELOCITY/3(Az_ec) -> Sum12/2  "Az_ec"
  INTERNAL REFERENCE MODEL VELOCITY/4(Vx_ref) -> ERROR CONTROLLER VELOCITY/1(Vx_ref)  "Vx_ref"
  ERROR CONTROLLER VELOCITY/1(Ax_ec) -> Sum6/2  "Ax_ec"
  ERROR CONTROLLER VELOCITY/2(Ay_ec) -> Sum7/2  "Ay_ec"
  Demux5/1 -> Sum16/1
  Sum12/1 -> Sum19/1
  [dv_outer] -> MatrixMultiply1/2
  Sum17/1 -> Vector Concatenate3/1  "dv_x"
  [Ay_f] -> Sum18/2
  [T_f] -> MATLAB Function1/1(T)
  INTERNAL REFERENCE MODEL VELOCITY/6(Vz_ref) -> ERROR CONTROLLER VELOCITY/3(Vz_ref)  "Vz_ref"
  [Az_f] -> Sum19/2
  Constant4/1 -> Sum21/1
  [phi_f] -> Sum15/2, MATLAB Function1/2(Phi)
  [theta_f] -> Sum21/2, MATLAB Function1/3(Theta)
  Sum16/1 -> [Theta_cmd]  "theta_cmd"
  [Theta_cmd] -> Saturation1/1
  [psi_traj] -> INTERNAL REFERENCE MODEL ATTITUDE/3(psi_cmd)
  [Phi_cmd] -> Saturation/1
  Saturation1/1 -> INTERNAL REFERENCE MODEL ATTITUDE/2(theta_cmd)  "theta_cmd"
  Saturation/1 -> INTERNAL REFERENCE MODEL ATTITUDE/1(phi_cmd)  "phi_cmd"
  Saturation4/1 -> Discrete Transfer Fcn/1
  Demux/4 -> Motor_4_omega_input/1
  Pseudoinverse2/1 -> Matrix Multiply/1
  Vector Concatenate2/1 -> Matrix Multiply/2
  Constant9/1 -> G2_comp/1(G2)
  Sum/1 -> Vector Concatenate2/3
  Demux1/3 -> Sum/1
  Demux1/2 -> Vector Concatenate2/2
  Constant2/1 -> G1+G2/1(G1)
  Discrete Transfer Fcn/1 -> G2_comp/2(domega)
  Constant3/1 -> G1+G2/2(G2)
  Demux/3 -> Motor_3_omega_input/1
  [omega_1_f] -> Vector Concatenate1/1
  Vector Concatenate1/1 -> G1+G2/3(omega), Sum8/2  "u"
  G2_comp/1(G2_comp) -> Sum/2  "G2_comp"
  Demux1/4 -> Vector Concatenate2/4
  Demux1/1 -> Vector Concatenate2/1
  Matrix Multiply/1 -> Saturation4/1, Sum8/1  "du"
  Demux/1 -> Motor_1_omega_input/1
  [omega_3_f] -> Vector Concatenate1/3
  Sum8/1 -> Demux/1  "u_cmd"
  Demux/2 -> Motor_2_omega_input/1
  [omega_2_f] -> Vector Concatenate1/2
  G1+G2/1(B_inner) -> Pseudoinverse2/1, Display/1  "B_inner"
  [dv_inner] -> Demux1/1  "dv_inner"
  [omega_4_f] -> Vector Concatenate1/4

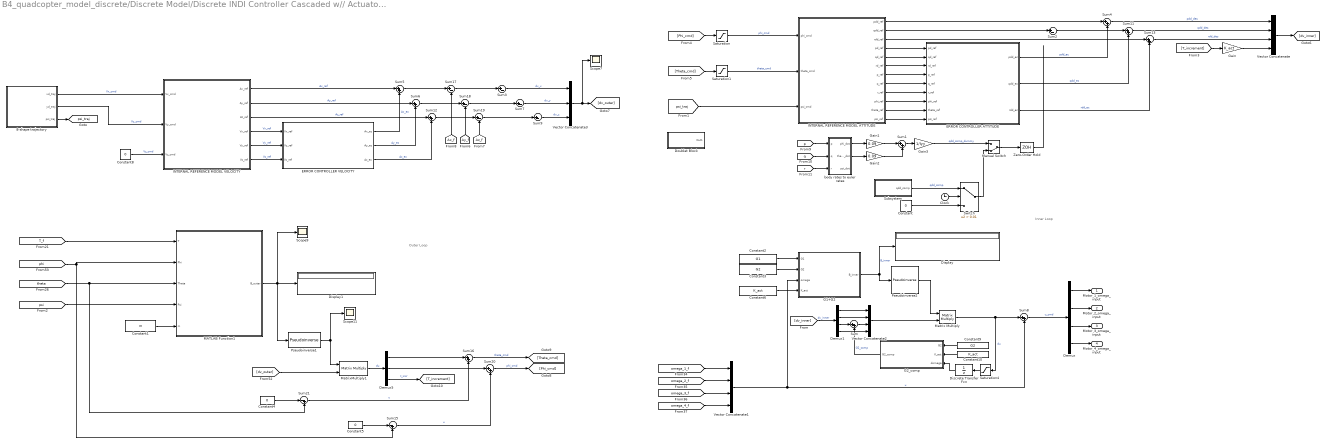
== system B4_quadcopter_model_discrete/Discrete Model/Discrete INDI Controller Cascaded w// Actuator Compensation ==
  note: Inner Loop
  note: Outer Loop
  8-shape trajectory : Subsystem
  Clock : Clock
  Constant : Constant  Value=0  SampleTime=sampling_time
  Constant1 : Constant  Value=m  SampleTime=sampling_time
  Constant10 : Constant  Value=K_act  SampleTime=sampling_time
  Constant2 : Constant  Value=G1  SampleTime=sampling_time
  Constant3 : Constant  Value=G2  SampleTime=sampling_time
  Constant4 : Constant  Value=0
  Constant5 : Constant  Value=0
  Constant6 : Constant  Value=K_act  SampleTime=sampling_time
  Constant8 : Constant  Value=0  SampleTime=sampling_time
  Constant9 : Constant  Value=G2  SampleTime=sampling_time
  Demux : Demux
  Demux1 : Demux
  Demux5 : Demux  Outputs=3
  Discrete Transfer Fcn : DiscreteTransferFcn  Denominator=[1 0]
  Display : Display
  Display1 : Display
  Doublet Block : Subsystem
  ERROR CONTROLLER ATTITUDE : Subsystem
  ERROR CONTROLLER VELOCITY : Subsystem
  G1+G2 : MATLAB Function  TreatAsAtomicUnit=on
  G2_comp : MATLAB Function  TreatAsAtomicUnit=on
  Gain : Gain  Gain=K_act
  Gain1 : Gain  Gain=0.09
  Gain2 : Gain  Gain=0.09
  Gain3 : Gain  Gain=1/Iyy
  INTERNAL REFERENCE MODEL ATTITUDE : Subsystem
  INTERNAL REFERENCE MODEL VELOCITY : Subsystem
  MATLAB Function1 : MATLAB Function  TreatAsAtomicUnit=on
  Manual Switch : ManualSwitch  CurrentSetting=0
  Matrix Multiply : Product  Multiplication=Matrix(*)
  MatrixMultiply1 : Product  Multiplication=Matrix(*)
  Pseudoinverse1 : dspinverses/Pseudoinverse  wanterr=off  SimulateUsing=Interpreted execution
      settings: SourceProductBaseCode=DS
  Pseudoinverse2 : dspinverses/Pseudoinverse  wanterr=off  SimulateUsing=Interpreted execution
      settings: SourceProductBaseCode=DS
  Saturation : Saturate
  Saturation1 : Saturate
  Saturation4 : Saturate  UpperLimit=12000  LowerLimit=10
  Scope11 : Scope
  Scope7 : Scope
  Scope9 : Scope
  Subsystem : Subsystem
  Sum{,1,4..6,8,11..13,16,20} (11 alike) : Sum  Inputs=|++
  Sum15 : Sum  Inputs=|-+
  Sum{2..3,7,9,17..19} (7 alike) : Sum  Inputs=|+-
  Sum21 : Sum  Inputs=|-+
  Switch : Switch  Criteria=u2 > Threshold  Threshold=0.01
  Vector Concatenate : Concatenate  NumInputs=4
  Vector Concatenate1 : Concatenate  NumInputs=4
  Vector Concatenate2 : Concatenate  NumInputs=4
  Vector Concatenate3 : Concatenate  NumInputs=3
  Zero-Order Hold : ZeroOrderHold  SampleTime=sampling_time
  body rates to euler rates : Subsystem
  Motor_1_omega_input : Outport
  Motor_2_omega_input : Outport  Port=2
  Motor_3_omega_input : Outport  Port=3
  Motor_4_omega_input : Outport  Port=4
  tag scope: psi_traj=global
  wires:
  G1+G2/1(B_inner) -> Pseudoinverse2/1, Display/1  "B_inner"
  Vector Concatenate1/1 -> G1+G2/3(omega), Sum8/2  "u"
  Vector Concatenate/1 -> [dv_inner]
  Matrix Multiply/1 -> Saturation4/1, Sum8/1  "du"
  Demux/1 -> Motor_1_omega_input/1
  [omega_4_f] -> Vector Concatenate1/4
  [omega_2_f] -> Vector Concatenate1/2
  Demux/3 -> Motor_3_omega_input/1
  Sum8/1 -> Demux/1  "u_cmd"
  Pseudoinverse2/1 -> Matrix Multiply/1
  [omega_1_f] -> Vector Concatenate1/1
  Demux/2 -> Motor_2_omega_input/1
  Demux/4 -> Motor_4_omega_input/1
  [omega_3_f] -> Vector Concatenate1/3
  INTERNAL REFERENCE MODEL VELOCITY/5(Vy_ref) -> ERROR CONTROLLER VELOCITY/2(Vy_ref)  "Vy_ref"
  Constant4/1 -> Sum21/1
  Sum16/1 -> [Theta_cmd]  "theta_cmd"
  Sum9/1 -> Vector Concatenate3/3  "dv_z"
  INTERNAL REFERENCE MODEL VELOCITY/2(Ay_ref) -> Sum6/1  "Ay_ref"
  Sum21/1 -> Sum16/2  "u"
  INTERNAL REFERENCE MODEL VELOCITY/6(Vz_ref) -> ERROR CONTROLLER VELOCITY/3(Vz_ref)  "Vz_ref"
  INTERNAL REFERENCE MODEL VELOCITY/4(Vx_ref) -> ERROR CONTROLLER VELOCITY/1(Vx_ref)  "Vx_ref"
  ERROR CONTROLLER VELOCITY/2(Ay_ec) -> Sum6/2  "Ay_ec"
  8-shape trajectory/1(xd_traj) -> INTERNAL REFERENCE MODEL VELOCITY/1(Vx_cmd)  "Vx_cmd"
  Sum7/1 -> Vector Concatenate3/2  "dv_y"
  ERROR CONTROLLER VELOCITY/1(Ax_ec) -> Sum5/2  "Ax_ec"
  Sum3/1 -> Vector Concatenate3/1  "dv_x"
  ERROR CONTROLLER VELOCITY/3(Az_ec) -> Sum12/2  "Az_ec"
  Sum12/1 -> Sum19/1
  Constant8/1 -> INTERNAL REFERENCE MODEL VELOCITY/3(Vz_cmd)  "Vz_cmd"
  Pseudoinverse1/1 -> Scope11/1, MatrixMultiply1/1
  Sum15/1 -> Sum20/2  "u"
  Vector Concatenate3/1 -> Scope7/1, [dv_outer]
  INTERNAL REFERENCE MODEL VELOCITY/1(Ax_ref) -> Sum5/1  "Ax_ref"
  INTERNAL REFERENCE MODEL VELOCITY/3(Az_ref) -> Sum12/1  "Az_ref"
  Sum20/1 -> [Phi_cmd]  "phi_cmd"
  [T_f] -> MATLAB Function1/1(T)
  Sum6/1 -> Sum18/1
  Constant5/1 -> Sum15/1
  [dv_outer] -> MatrixMultiply1/2
  MATLAB Function1/1(B_outer) -> Scope9/1, Display1/1, Pseudoinverse1/1
  Demux5/3 -> [T_increment]  "t_incr"
  MatrixMultiply1/1 -> Demux5/1  "du"
  8-shape trajectory/2(yd_traj) -> INTERNAL REFERENCE MODEL VELOCITY/2(Vy_cmd)  "Vy_cmd"
  [T_increment] -> Gain/1
  [Ax_f] -> Sum17/2
  [Ay_f] -> Sum18/2
  [Az_f] -> Sum19/2
  [Phi_cmd] -> Saturation/1
  [theta] -> Sum21/2, MATLAB Function1/3(Theta)
  [phi] -> Sum15/2, MATLAB Function1/2(Phi)
  INTERNAL REFERENCE MODEL ATTITUDE/4(pd_ref) -> ERROR CONTROLLER ATTITUDE/1(pd_ref)
  INTERNAL REFERENCE MODEL ATTITUDE/7(p_ref) -> ERROR CONTROLLER ATTITUDE/4(p_ref)
  ERROR CONTROLLER ATTITUDE/3(rdd_ec) -> Sum13/2  "rdd_ec"
  ERROR CONTROLLER ATTITUDE/2(qdd_ec) -> Sum11/2  "qdd_ec"
  INTERNAL REFERENCE MODEL ATTITUDE/5(qd_ref) -> ERROR CONTROLLER ATTITUDE/2(qd_ref)
  INTERNAL REFERENCE MODEL ATTITUDE/11(theta_ref) -> ERROR CONTROLLER ATTITUDE/8(theta_ref)
  INTERNAL REFERENCE MODEL ATTITUDE/1(pdd_ref) -> Sum4/1
  INTERNAL REFERENCE MODEL ATTITUDE/3(rdd_ref) -> Sum13/1
  INTERNAL REFERENCE MODEL ATTITUDE/8(q_ref) -> ERROR CONTROLLER ATTITUDE/5(q_ref)
  ERROR CONTROLLER ATTITUDE/1(pdd_ec) -> Sum4/2  "pdd_ec"
  INTERNAL REFERENCE MODEL ATTITUDE/6(rd_ref) -> ERROR CONTROLLER ATTITUDE/3(rd_ref)
  INTERNAL REFERENCE MODEL ATTITUDE/2(qdd_ref) -> Sum2/1
  INTERNAL REFERENCE MODEL ATTITUDE/10(phi_ref) -> ERROR CONTROLLER ATTITUDE/7(phi_ref)
  INTERNAL REFERENCE MODEL ATTITUDE/12(psi_ref) -> ERROR CONTROLLER ATTITUDE/9(psi_ref)
  INTERNAL REFERENCE MODEL ATTITUDE/9(r_ref) -> ERROR CONTROLLER ATTITUDE/6(r_ref)
  Sum13/1 -> Vector Concatenate/3  "rdd_des"
  Sum4/1 -> Vector Concatenate/1  "pdd_des"
  Sum11/1 -> Vector Concatenate/2  "qdd_des"
  Gain/1 -> Vector Concatenate/4
  Constant3/1 -> G1+G2/2(G2)
  Constant6/1 -> G1+G2/4(K_act)
  Constant2/1 -> G1+G2/1(G1)
  Constant9/1 -> G2_comp/1(G2)
  Constant10/1 -> G2_comp/2(K_act)
  Discrete Transfer Fcn/1 -> G2_comp/3(domega)
  [dv_inner] -> Demux1/1  "dv_inner"
  Sum/1 -> Vector Concatenate2/3
  Demux1/3 -> Sum/1
  Demux1/2 -> Vector Concatenate2/2
  Demux1/1 -> Vector Concatenate2/1
  Demux1/4 -> Vector Concatenate2/4
  Vector Concatenate2/1 -> Matrix Multiply/2
  G2_comp/1(G2_comp) -> Sum/2  "G2_comp"
  Sum5/1 -> Sum17/1
  Sum2/1 -> Sum11/1
  8-shape trajectory/3(psi_traj) -> [psi_traj]
  [Theta_cmd] -> Saturation1/1
  Saturation4/1 -> Discrete Transfer Fcn/1
  Saturation/1 -> INTERNAL REFERENCE MODEL ATTITUDE/1(phi_cmd)  "phi_cmd"
  Sum17/1 -> Sum3/1
  Sum18/1 -> Sum7/1
  Sum19/1 -> Sum9/1
  Constant1/1 -> MATLAB Function1/5(m)
  Demux5/2 -> Sum20/1
  Demux5/1 -> Sum16/1
  [psi] -> MATLAB Function1/4(Psi)
  Gain3/1 -> Manual Switch/1  "qdd_comp_dummy"
  [p] -> body rates to euler rates/1(p)
  [q] -> body rates to euler rates/2(q)
  [r] -> body rates to euler rates/3(r)
  body rates to euler rates/1(phi_dot) -> Gain1/1
  body rates to euler rates/2(theta_dot) -> Gain2/1
  Gain1/1 -> Sum1/1
  Gain2/1 -> Sum1/2
  Sum1/1 -> Gain3/1
  Subsystem/1(qdd_comp) -> Switch/1  "qdd_comp"
  Manual Switch/1 -> Zero-Order Hold/1
  Clock/1 -> Switch/2
  Constant/1 -> Switch/3
  Switch/1 -> Manual Switch/2
  Zero-Order Hold/1 -> ?
  Saturation1/1 -> INTERNAL REFERENCE MODEL ATTITUDE/2(theta_cmd)  "theta_cmd"
  [psi_traj] -> INTERNAL REFERENCE MODEL ATTITUDE/3(psi_cmd)
